simulink model "AudioDeviceReader_BasicModel"  (R2019b)
settings: Solver=FixedStepDiscrete  StartTime=0.0  StopTime=inf  RelTol=1e-3
libraries: audiosources x1, dspsnks4 x1
settings Model: Creator=The MathWorks, Inc.  LastModifiedBy=adi
settings SolverCC: AutoInsertRateTranBlk=on
settings DataIOCC: LimitDataPoints=on  SaveOutput=off  SignalLogging=off  SaveTime=off  ReturnWorkspaceOutputs=off
settings OptimizationCC: LifeSpan=inf
settings DebuggingCC: AlgebraicLoopMsg=error  SingleTaskRateTransMsg=error  AllowSymbolicDim=off  SFUnexpectedBacktrackingDiag=warning  SFNoUnconditionalDefaultTransitionDiag=warning  SFExecutionAtInitializationDiag=none  ArithmeticOperatorsInVariantConditions=warning
settings SFSimCC: SimUseLocalCustomCode=off  CustomCodeUndefinedFunction=UseInterfaceOnly
settings RTWCC: RTWUseLocalCustomCode=off
settings CodeAppCC: StateflowObjectComments=on
settings GRTTargetCC: TargetLangStandard=C89/C90 (ANSI)  GeneratePreprocessorConditionals=Disable all
settings ConfigComp: CovMetricSettings=dw  CovHtmlReporting=on  CovSaveCumulativeToWorkspaceVar=on  CovSaveSingleToWorkspaceVar=on  CovShowResultsExplorer=off  CovExternalEMLEnable=off  CovSFcnEnable=off

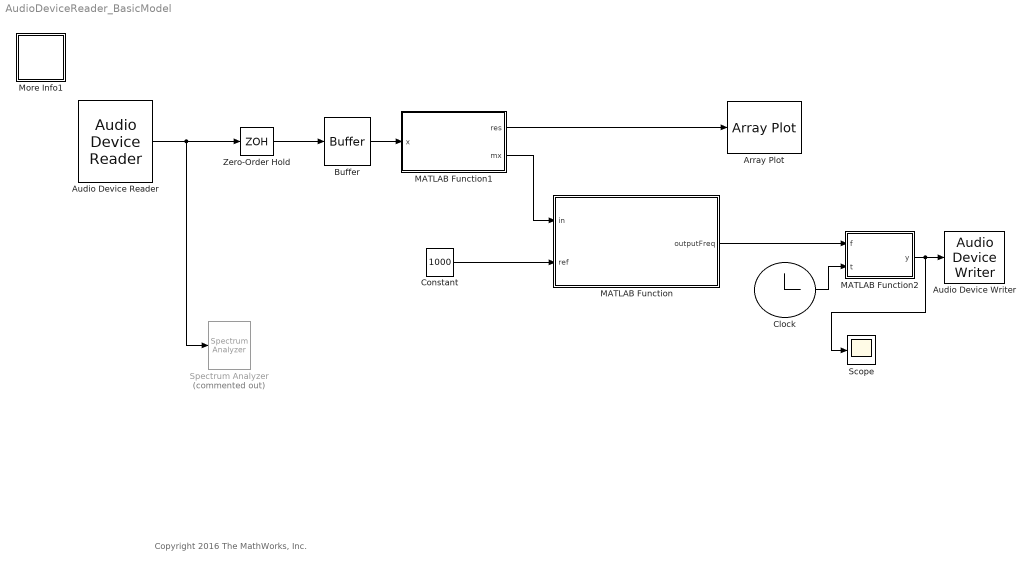
== system AudioDeviceReader_BasicModel ==
  note: Copyright 2016 The MathWorks, Inc.
  Array Plot : ArrayPlot
  Audio Device Reader : audiosources/Audio Device Reader  Driver=CoreAudio  Device=MacBook Pro Microphone  SampleRate=44100  NumChannels=1  SamplesPerFrame=1024  BitDepth=16-bit integer  NumBuffers=10  DefaultInputChannelMapping=on  InputChannelMapping=1:2  OutputNumOverrunSamples=off  OutputDataType=double  DriverIdx=5  DeviceWarnFlag=''
      settings: SourceProductName=Audio Toolbox  SourceProductBaseCode=AU
  Audio Device Writer : dspsnks4/Audio Device Writer  Driver=CoreAudio  Device=MacBook Pro Speakers  InheritSampleRate=off  SampleRate=2000  BitDepth=16-bit integer  BufferSize=4096  NumBuffers=10  DefaultOutputChannelMapping=on  OutputChannelMapping=1:2  OutputNumUnderrunSamples=off  DriverIdx=5  DeviceWarnFlag=''
  Buffer : Buffer  N=1024  OutputFrames=off
  Clock : Clock
  Constant : Constant  Value=1000
  MATLAB Function : MATLAB Function  TreatAsAtomicUnit=on
  MATLAB Function1 : MATLAB Function  TreatAsAtomicUnit=on
  MATLAB Function2 : MATLAB Function  TreatAsAtomicUnit=on
  More Info1 : Subsystem
      settings: OpenFcn=web(fullfile(docroot, 'audio/ref/audiodevicereader.html'))
      mask Display: disp('?')
  Scope : Scope
  Spectrum Analyzer : SpectrumAnalyzer  Commented=on
  Zero-Order Hold : ZeroOrderHold  SampleTime=-1
  wires:
  Audio Device Reader/1 -> Zero-Order Hold/1, Spectrum Analyzer/1
  Zero-Order Hold/1 -> Buffer/1
  Buffer/1 -> MATLAB Function1/1(x)
  MATLAB Function1/1(res) -> Array Plot/1
  MATLAB Function1/2(mx) -> MATLAB Function/1(in)
  Constant/1 -> MATLAB Function/2(ref)
  Clock/1 -> MATLAB Function2/2(t)
  MATLAB Function2/1(y) -> Scope/1, Audio Device Writer/1
  MATLAB Function/1(outputFreq) -> MATLAB Function2/1(f)

== system AudioDeviceReader_BasicModel/More Info1 ==

== matlab function AudioDeviceReader_BasicModel/MATLAB Function1 ==
  data: res output; mx output; x input
function [res,mx ] = fcn(x)
Fs = 96000;
xdft = fft(x);
fftabs = abs(xdft(1:length(x)/2+1));
freq = 0:Fs/length(x):(Fs/2);
[~,maxindex] = max(fftabs);
mx = freq(maxindex);
res = fftabs;
mx = mx/2;
fprintf('The maximum occurs at %2.1f Hz\n',mx );
end

== matlab function AudioDeviceReader_BasicModel/MATLAB Function ==
  data: in input; ref input; outputFreq output
function outputFreq = fcn(in,ref)
margin = 0;
if (in > ref + margin)
    outputFreq = 50;
else
    outputFreq = 0;
    
% elseif (in < ref - margin)
%     outputFreq = 350;
% else
%     outputFreq = 200;
% end

end

== matlab function AudioDeviceReader_BasicModel/MATLAB Function2 ==
  data: f input; y output; t input
function y = fcn(f,t)
A = 5;
y = A*sin(f*t);
